simulink model "aufgabe23A"  (R2014a)
settings: Solver=ode45  StartTime=0.0  StopTime=10.0  RelTol=1e-3
settings Model: Creator=s55812  LastModifiedBy=s55812

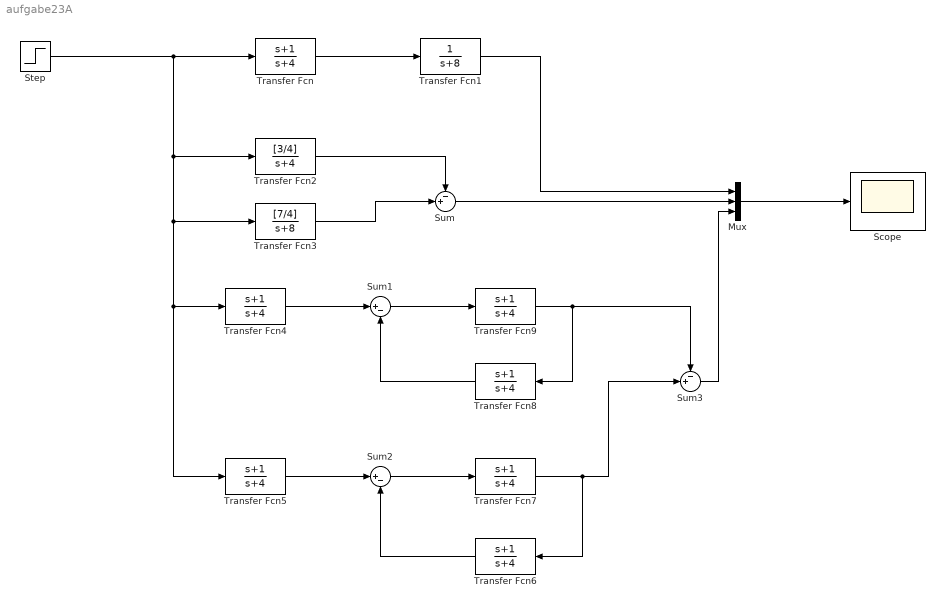
== system aufgabe23A ==
  Mux : Mux  Inputs=3
  Scope : Scope
  Step : Step  SampleTime=0
  Sum : Sum  Inputs=-+|
  Sum1 : Sum  Inputs=|+-
  Sum2 : Sum  Inputs=|+-
  Sum3 : Sum  Inputs=-+|
  Transfer Fcn{,4..9} (7 alike) : TransferFcn  Numerator=[1 1]  Denominator=[1 4]
  Transfer Fcn1 : TransferFcn  Denominator=[1 8]
  Transfer Fcn2 : TransferFcn  Numerator=[3/4]  Denominator=[1 4]
  Transfer Fcn3 : TransferFcn  Numerator=[7/4]  Denominator=[1 8]
  wires:
  Mux/1 -> Scope/1
  Step/1 -> Transfer Fcn5/1, Transfer Fcn4/1, Transfer Fcn3/1, Transfer Fcn2/1, Transfer Fcn/1
  Transfer Fcn/1 -> Transfer Fcn1/1
  Transfer Fcn1/1 -> Mux/1
  Transfer Fcn2/1 -> Sum/1
  Transfer Fcn3/1 -> Sum/2
  Sum/1 -> Mux/2
  Transfer Fcn4/1 -> Sum1/1
  Transfer Fcn5/1 -> Sum2/1
  Sum1/1 -> Transfer Fcn9/1
  Sum2/1 -> Transfer Fcn7/1
  Transfer Fcn7/1 -> Transfer Fcn6/1, Sum3/2
  Transfer Fcn9/1 -> Transfer Fcn8/1, Sum3/1
  Transfer Fcn8/1 -> Sum1/2
  Transfer Fcn6/1 -> Sum2/2
  Sum3/1 -> Mux/3
